simulink model "Impedance"  (R2020b)
settings: Solver=FixedStepAuto  StartTime=0.0  StopTime=5  FixedStep=0.005  RelTol=1e-3
values from neighbouring files (symbols this model uses):
  inv_Md = inv(Md)    [params.m]
  Kd = diag([30 30 14 1 1 1])    [params.m]
  Kp = diag([300 1000 300 1 1 1])    [params.m]
  Md = diag([1 0.1 1 1 1 1])    [params.m]
libraries: robotcorelib x1, vrlib x1
settings Model: Creator=andre  LastModifiedBy=filippo

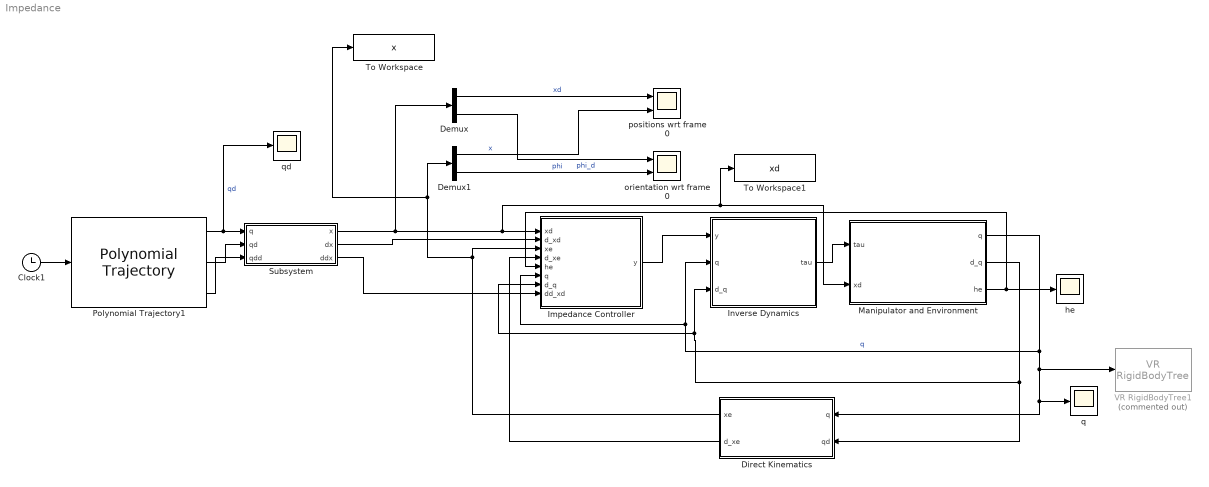
== system Impedance ==
  Clock1 : Clock
  Demux : Demux  Outputs=2
  Demux1 : Demux  Outputs=2
  Direct Kinematics : Subsystem
  Impedance Controller : Subsystem
  Inverse Dynamics : Subsystem
  Manipulator and Environment : Subsystem
  Polynomial Trajectory1 : robotcorelib/Polynomial Trajectory  WaypointSource=Internal  Waypoints=[0,0,0.05;0,0,-0.1;0,0.1,0.1]  TimePoints=[ 0, 2, 4 ]  TimeInterval=[ 1, 4 ]  Method=Cubic Polynomial  ParameterSource=Internal  VelocityBoundaryCondition=zeros(3,3)  AccelerationBoundaryCondition=zeros( 2, 5 )  SimulateUsing=Interpreted execution
  Subsystem : Subsystem
  To Workspace : ToWorkspace  VariableName=x  SaveFormat=Timeseries  SampleTime=-1
  To Workspace1 : ToWorkspace  VariableName=xd  SaveFormat=Timeseries  SampleTime=-1
  VR RigidBodyTree1 : vrlib/VR RigidBodyTree  Commented=on  RBT=robot  useRBT=on  Ts=-1  ForceViewerOpen=on
      settings: SourceProductBaseCode=SL
  he : Scope
  orientation wrt frame 0 : Scope  NumInputPorts=2
  positions wrt frame 0 : Scope  NumInputPorts=2
  q : Scope
  qd : Scope
  wires:
  Impedance Controller/1(y) -> Inverse Dynamics/1(y)
  Manipulator and Environment/2(d_q) -> Direct Kinematics/2(qd), Inverse Dynamics/3(d_q), Impedance Controller/7(d_q)
  Direct Kinematics/2(d_xe) -> Impedance Controller/4(d_xe)
  Manipulator and Environment/3(he) -> he/1, Impedance Controller/5(he)
  Direct Kinematics/1(xe) -> Impedance Controller/3(xe), To Workspace/1, Demux1/1
  Inverse Dynamics/1(tau) -> Manipulator and Environment/1(tau)
  Subsystem/1(x) -> Demux/1, To Workspace1/1, Manipulator and Environment/2(xd), Impedance Controller/1(xd)
  Subsystem/2(dx) -> Impedance Controller/2(d_xd)
  Polynomial Trajectory1/1 -> Subsystem/1(q), qd/1  "qd"
  Clock1/1 -> Polynomial Trajectory1/1
  Demux1/1 -> positions wrt frame 0/2  "x"
  Demux/1 -> positions wrt frame 0/1  "xd"
  Demux/2 -> orientation wrt frame 0/1  "phi_d"
  Demux1/2 -> orientation wrt frame 0/2  "phi"
  Manipulator and Environment/1(q) -> VR RigidBodyTree1/1, q/1, Direct Kinematics/1(q), Inverse Dynamics/2(q), Impedance Controller/6(q)  "q"
  Subsystem/3(ddx) -> Impedance Controller/8(dd_xd)
  Polynomial Trajectory1/2 -> Subsystem/2(qd)
  Polynomial Trajectory1/3 -> Subsystem/3(qdd)

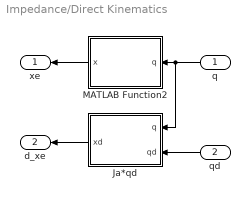
== system Impedance/Direct Kinematics ==
  q : Inport
  qd : Inport  Port=2
  Ja*qd : MATLAB Function  TreatAsAtomicUnit=on
  MATLAB Function2 : MATLAB Function  TreatAsAtomicUnit=on
  xe : Outport
  d_xe : Outport  Port=2
  wires:
  Ja*qd/1(xd) -> d_xe/1
  MATLAB Function2/1(x) -> xe/1
  q/1 -> Ja*qd/1(q), MATLAB Function2/1(q)
  qd/1 -> Ja*qd/2(qd)

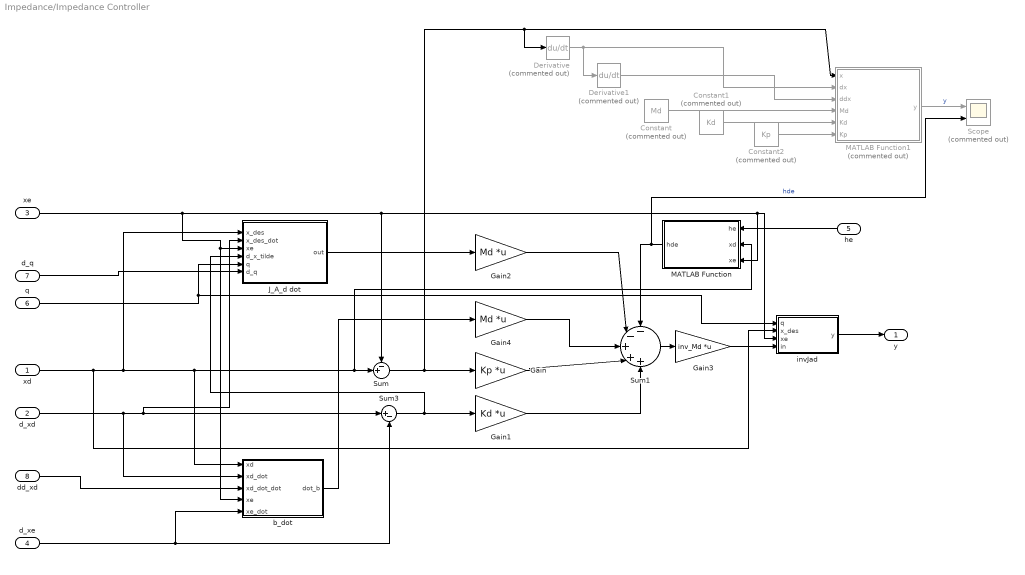
== system Impedance/Impedance Controller ==
  xd : Inport
  d_xd : Inport  Port=2
  xe : Inport  Port=3
  d_xe : Inport  Port=4
  he : Inport  Port=5
  q : Inport  Port=6
  d_q : Inport  Port=7
  dd_xd : Inport  Port=8
  Constant : Constant  Commented=on  Value=Md
  Constant1 : Constant  Commented=on  Value=Kd
  Constant2 : Constant  Commented=on  Value=Kp
  Derivative : Derivative  Commented=on
  Derivative1 : Derivative  Commented=on
  Gain : Gain  Gain=Kp  Multiplication=Matrix(K*u)
  Gain1 : Gain  Gain=Kd  Multiplication=Matrix(K*u)
  Gain2 : Gain  Gain=Md  Multiplication=Matrix(K*u)
  Gain3 : Gain  Gain=inv_Md  Multiplication=Matrix(K*u)
  Gain4 : Gain  Gain=Md  Multiplication=Matrix(K*u)
  J_A_d dot : MATLAB Function  TreatAsAtomicUnit=on
  MATLAB Function : MATLAB Function  TreatAsAtomicUnit=on
  MATLAB Function1 : MATLAB Function  Commented=on  TreatAsAtomicUnit=on
  Scope : Scope  Commented=on  NumInputPorts=2
  Sum : Sum  Inputs=-+|
  Sum1 : Sum  Inputs=-|-|+|+|+
  Sum3 : Sum  Inputs=|+-
  b_dot : MATLAB Function  TreatAsAtomicUnit=on
  invJad : MATLAB Function  TreatAsAtomicUnit=on
  y : Outport
  wires:
  xd/1 -> invJad/2(x_des), Sum/2, MATLAB Function/2(xd), b_dot/1(xd), J_A_d dot/1(x_des)
  xe/1 -> invJad/3(xe), MATLAB Function/3(xe), Sum/1, b_dot/4(xe), J_A_d dot/3(xe)
  Gain1/1 -> Sum1/5
  Gain/1 -> Sum1/4
  d_xe/1 -> b_dot/5(xe_dot), Sum3/2
  d_xd/1 -> b_dot/2(xd_dot), J_A_d dot/2(x_des_dot), Sum3/1
  Gain3/1 -> invJad/4(in)
  q/1 -> J_A_d dot/5(q), invJad/1(q)
  Sum1/1 -> Gain3/1
  he/1 -> MATLAB Function/1(he)
  MATLAB Function/1(hde) -> Scope/2, Sum1/1  "hde"
  Gain4/1 -> Sum1/3
  d_q/1 -> J_A_d dot/6(d_q)
  b_dot/1(dot_b) -> Gain4/1
  J_A_d dot/1(out) -> Gain2/1
  Gain2/1 -> Sum1/2
  invJad/1(y) -> y/1
  dd_xd/1 -> b_dot/3(xd_dot_dot)
  MATLAB Function1/1(y) -> Scope/1  "y"
  Constant/1 -> MATLAB Function1/4(Md)
  Constant1/1 -> MATLAB Function1/5(Kd)
  Constant2/1 -> MATLAB Function1/6(Kp)
  Sum/1 -> Derivative/1, MATLAB Function1/1(x), Gain/1
  Sum3/1 -> Gain1/1, J_A_d dot/4(d_x_tilde)
  Derivative/1 -> Derivative1/1, MATLAB Function1/2(dx)
  Derivative1/1 -> MATLAB Function1/3(ddx)

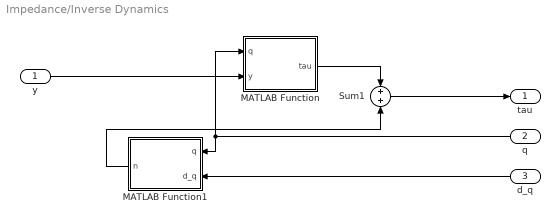
== system Impedance/Inverse Dynamics ==
  y : Inport
  q : Inport  Port=2
  d_q : Inport  Port=3
  MATLAB Function : MATLAB Function  TreatAsAtomicUnit=on
  MATLAB Function1 : MATLAB Function  TreatAsAtomicUnit=on
  Sum1 : Sum
  tau : Outport
  wires:
  MATLAB Function1/1(n) -> Sum1/2
  d_q/1 -> MATLAB Function1/2(d_q)
  q/1 -> MATLAB Function1/1(q), MATLAB Function/1(q)
  y/1 -> MATLAB Function/2(y)
  MATLAB Function/1(tau) -> Sum1/1
  Sum1/1 -> tau/1

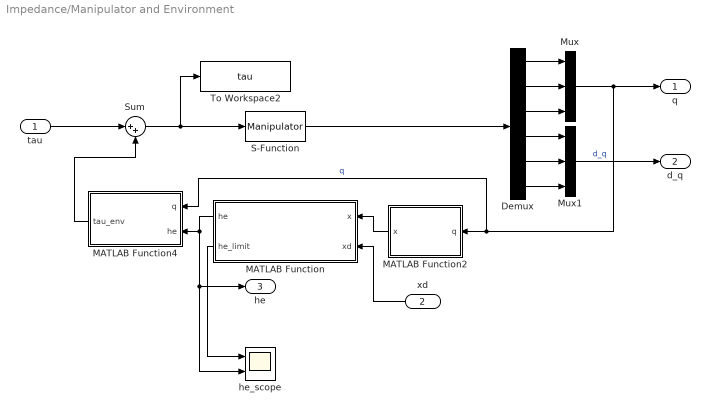
== system Impedance/Manipulator and Environment ==
  tau : Inport
  xd : Inport  Port=2
  Demux : Demux  Outputs=6
  MATLAB Function : MATLAB Function  TreatAsAtomicUnit=on
  MATLAB Function2 : MATLAB Function  TreatAsAtomicUnit=on
  MATLAB Function4 : MATLAB Function  TreatAsAtomicUnit=on
  Mux : Mux  Inputs=3
  Mux1 : Mux  Inputs=3
  S-Function : S-Function  FunctionName=Manipulator  Parameters=param  SFunctionDeploymentMode=off  EnableBusSupport=off
  Sum : Sum  Inputs=|++
  To Workspace2 : ToWorkspace  VariableName=tau  SaveFormat=Timeseries  SampleTime=-1
  he_scope : Scope  NumInputPorts=2
  q : Outport
  d_q : Outport  Port=2
  he : Outport  Port=3
  wires:
  Demux/4 -> Mux1/1
  tau/1 -> Sum/1
  Demux/3 -> Mux/3
  Demux/1 -> Mux/1
  Demux/5 -> Mux1/2
  Demux/6 -> Mux1/3
  Demux/2 -> Mux/2
  Mux1/1 -> d_q/1  "d_q"
  Mux/1 -> q/1, MATLAB Function4/1(q), MATLAB Function2/1(q)  "q"
  MATLAB Function2/1(x) -> MATLAB Function/1(x)
  S-Function/1 -> Demux/1
  Sum/1 -> To Workspace2/1, S-Function/1
  MATLAB Function/1(he) -> he_scope/2, he/1, MATLAB Function4/2(he)
  MATLAB Function4/1(tau_env) -> Sum/2
  MATLAB Function/2(he_limit) -> he_scope/1
  xd/1 -> MATLAB Function/2(xd)

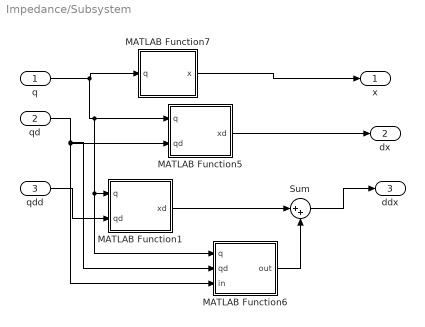
== system Impedance/Subsystem ==
  q : Inport
  qd : Inport  Port=2
  qdd : Inport  Port=3
  MATLAB Function1 : MATLAB Function  TreatAsAtomicUnit=on
  MATLAB Function5 : MATLAB Function  TreatAsAtomicUnit=on
  MATLAB Function6 : MATLAB Function  TreatAsAtomicUnit=on
  MATLAB Function7 : MATLAB Function  TreatAsAtomicUnit=on
  Sum : Sum  Inputs=|++
  x : Outport
  dx : Outport  Port=2
  ddx : Outport  Port=3
  wires:
  q/1 -> MATLAB Function6/1(q), MATLAB Function1/1(q), MATLAB Function5/1(q), MATLAB Function7/1(q)
  MATLAB Function7/1(x) -> x/1
  MATLAB Function5/1(xd) -> dx/1
  qdd/1 -> MATLAB Function1/2(qd)
  qd/1 -> MATLAB Function6/3(in), MATLAB Function5/2(qd), MATLAB Function6/2(qd)
  MATLAB Function6/1(out) -> Sum/2
  MATLAB Function1/1(xd) -> Sum/1
  Sum/1 -> ddx/1

== matlab function Impedance/Direct Kinematics/MATLAB Function2 ==
  data: q input; x output; param parameter
function x = Kin(q,param)
    x = Kinematics(q,param);
end

== matlab function Impedance/Direct Kinematics/Ja*qd ==
  data: q input; xd output; qd input; param parameter
function xd = Ja(q, qd, param)
    Ja = AnalyticalJacobian(q,param);
    xd = Ja * qd;
end

== matlab function Impedance/Impedance Controller/J_A_d dot ==
  data: x_des input; x_des_dot input; out output; xe input; d_x_tilde input; q input; d_q input; param parameter
function out = dot_Jad(x_des, x_des_dot, xe, d_x_tilde, q, d_q, param)    
    % Get euler angles from x_tilde
    x_tilde = x_des - xe;
    O_d_e = - x_tilde(4:6);
    phi = O_d_e(1);
    theta = O_d_e(2);
    
    % Get velocities along euler angles
    omega_d_e = - d_x_tilde(4:6);
    theta_dot = omega_d_e(1);
    phi_dot = omega_d_e(2);
    
    % Build rotation matrix
    Rd = eul2rotm(x_des(4:6)', 'ZYZ');
    R = [Rd', zeros(3,3); zeros(3,3), Rd'];
    
    % Get Ta and the necessary transformations
    Ta =  [1, 0, 0, 0, 0, 0;
            0, 1, 0, 0, 0, 0;
            0, 0, 1, 0, 0, 0;
            0, 0, 0, 0, -sin(phi), cos(phi) * sin(theta);
            0, 0, 0, 0, cos(phi), sin(phi) * sin(theta);
            0, 0, 0, 1, 0, cos(theta)];
    Ta_inv = pinv(Ta);
    
    % Precomputed dot inverse of Ta
    d_Ta = [[0, 0, 0, 0,                 0,                                                           0]
            [0, 0, 0, 0,                 0,                                                           0]
            [0, 0, 0, 0,                 0,                                                           0]
            [0, 0, 0, 0, -phi_dot*cos(phi), theta_dot*cos(phi)*cos(theta) - phi_dot*sin(phi)*sin(theta)]
            [0, 0, 0, 0, -phi_dot*sin(phi), phi_dot*cos(phi)*sin(theta) + theta_dot*cos(theta)*sin(phi)]
            [0, 0, 0, 0,                 0,                                       -theta_dot*sin(theta)]];
    Ta_inv_dot = pinv(d_Ta);
    
    % Build the skew symmetric matrix used to compute the derivative
    wd_d = x_des_dot(4:6);
    Swd = [   0      -wd_d(3)   wd_d(2);
              wd_d(3)       0      -wd_d(1);
             -wd_d(2)   wd_d(1)     0   ];
    
    % Compute the RS matrix with Rd' and the skew symmetric matrix
    RS = [Rd'*Swd, zeros(3,3); zeros(3,3), Rd'*Swd];
    
    % Jad = invTA*R*J
    dot_Jad = Ta_inv*(RS*Jacobian(q,param)+R*Jacobian_dot(q,d_q,param))+Ta_inv_dot*R*Jacobian(q,param);

    out = dot_Jad * d_q;
end

== matlab function Impedance/Impedance Controller/b_dot ==
  data: xd input; xd_dot input; xd_dot_dot input; dot_b output; xe input; xe_dot input
function dot_b = dot_b(xd, xd_dot, xd_dot_dot, xe, xe_dot)
    Rd = eul2rotm(xd(4:6)', 'ZYZ');
    
    % Get x_tilde and x_tilde_dot
    x_tilde = xd - xe;
    d_x_tilde = xd_dot - xe_dot;
    
    % Get angles from x_tilde
    phi_d_e = - x_tilde(4:6); 
    phi = phi_d_e(1);
    theta = phi_d_e(2);
    theta_dot = -d_x_tilde(2);
    phi_dot = -d_x_tilde(1);
    
    % Get the transformation matrix ZYZ
    T = [0   -sin(phi)  cos(phi)*sin(theta);
         0  cos(theta)  sin(phi)*sin(theta);
         1      0                cos(theta)];
    
    % Compute T_inv_dot
    d_T = [[0,     -phi_dot*cos(phi), theta_dot*cos(phi)*cos(theta) - phi_dot*sin(phi)*sin(theta)]
            [0, -theta_dot*sin(theta), phi_dot*cos(phi)*sin(theta) + theta_dot*cos(theta)*sin(phi)]
            [0,                     0,                                       -theta_dot*sin(theta)]];
    invT = pinv(T);
    invDT = -invT*d_T*invT;
            
    % Angular velocity and linearSwd_d velocity
    wd_d = xd_dot(4:6);
    dot_wd_d = xd_dot_dot(4:6);
    
    % Skew symmetric matrix
    Swd_d = [   0      -wd_d(3)   wd_d(2);
              wd_d(3)       0      -wd_d(1);
             -wd_d(2)   wd_d(1)     0   ];
    d_Rd = Rd'*Swd_d;
    
    % o d-e and its derivatives
    oe = xe(1:3);
    od = xd(1:3);
    dot_oe = xe_dot(1:3);
    dot_od = xd_dot(1:3);
    od_dot = xd_dot(1:3);
    od_dot_dot = xd_dot_dot(1:3);
    
    
    dot_b = [Rd'*od_dot_dot+d_Rd'*od_dot + cross(Rd'*dot_wd_d,Rd'*(od-oe)) + cross(Rd'*wd_d, Rd'*(dot_od-dot_oe));
        invDT*wd_d + invT*dot_wd_d];
end

== matlab function Impedance/Inverse Dynamics/MATLAB Function1 ==
  data: q input; n output; d_q input; param parameter
function n = n(q,d_q,param)
    % Compute C and G used in the model of n(q,d_q)
    C = double(C_Lagrangian(q, d_q, param));
    G = double(G_Lagrangian(q, param));
    Fsv = param.Fsv;

    n = C * d_q + G + Fsv * d_q;
end

== matlab function Impedance/Subsystem/MATLAB Function1 ==
  data: q input; qd input; xd output; param parameter
function xd = Ja(q, qd, param)
    Ja = AnalyticalJacobian(q,param);
    xd = Ja * qd;
end

== matlab function Impedance/Manipulator and Environment/MATLAB Function ==
  data: x input; xd input; he output; param parameter; he_limit output
function [he, he_limit] = environment(x, xd, param)
    if x(param.axis) >= param.wall 

        % set up the rest position frame
        xr = zeros(6,1);
        xr(param.axis) = param.wall;

        xe = zeros(6,1);
        xe(param.axis) = x(param.axis);

        he = param.K * (xe - xr);
        dx_rd = zeros(6,1);
        dx_rd(param.axis) = xd(param.axis) - xr(param.axis);
        % At the limit
        he_limit =  param.K/(eye(6) + param.K / param.Kp) * dx_rd;
    else
        he = zeros(6,1);
        he_limit = zeros(6,1);
    end
end

== matlab function Impedance/Manipulator and Environment/MATLAB Function2 ==
  data: q input; x output; param parameter
function x = Kin(q,param)
    x = Kinematics(q,param);
end

== matlab function Impedance/Subsystem/MATLAB Function5 ==
  data: q input; qd input; xd output; param parameter
function xd = Ja(q, qd, param)
    Ja = AnalyticalJacobian(q,param);
    xd = Ja * qd;
end

== matlab function Impedance/Subsystem/MATLAB Function6 ==
  data: q input; qd input; in input; out output; param parameter
function out = dot_Ja(q, qd, in, param)
    d_Ja = AnalyticalJacobian_dot(q,qd,param);
    out = d_Ja * in;
end

== matlab function Impedance/Subsystem/MATLAB Function7 ==
  data: q input; x output; param parameter
function x = Kin(q,param)
    x = Kinematics(q,param);
end

== matlab function Impedance/Manipulator and Environment/MATLAB Function4 ==
  data: q input; he input; tau_env output; param parameter
function tau_env = JT(q, he, param)
    tau_env = -Jacobian(q, param)' * he;
end

== matlab function Impedance/Impedance Controller/MATLAB Function1 ==
  data: x input; y output; dx input; ddx input; Md input; Kd input; Kp input
function y = eq(x, dx, ddx, Md, Kd, Kp)
    y = Md*ddx + Kd*dx + Kp*x;

== matlab function Impedance/Inverse Dynamics/MATLAB Function ==
  data: q input; y input; tau output; param parameter
function tau = B(q,y,param)
    B_matrix = B_Lagrangian(q, param);
    tau =  B_matrix * y;
end

== matlab function Impedance/Impedance Controller/invJad ==
  data: q input; x_des input; xe input; y output; in input; param parameter
function y = invJad(q, x_des, xe, in, param)
    x_tilde = x_des - xe;
    Rd = eul2rotm(-x_tilde(4:6)','ZYZ');
    angles = -x_tilde(4:6);
    
%     Compute Ta(phi_de) in this case ZYZ
    ph = -angles(1);
    th = -angles(2);
    Ta =   [1, 0, 0, 0, 0, 0;
            0, 1, 0, 0, 0, 0;
            0, 0, 1, 0, 0, 0;
            0, 0, 0, 0, -sin(ph), cos(ph) * sin(th);
            0, 0, 0, 0, cos(ph), sin(ph) * sin(th);
            0, 0, 0, 1, 0, cos(th)];
        
    Jad = pinv(Ta)*[Rd', zeros(3,3); zeros(3,3), Rd']*Jacobian(q, param);
 
    %Jad = AnalyticalJacobian(q,param);
     
    y = pinv(Jad) * in;
end

== matlab function Impedance/Impedance Controller/MATLAB Function ==
  data: he input; hde output; xd input; xe input
function hde = to_hde(he, xd, xe)
    hde = zeros(6,1);
    Rd_e = eul2rotm(((xd(4:6) - xe(4:6)))', 'ZYZ');
    
    hde(1:3) = Rd_e * he(1:3);
    hde(4:6) = Rd_e * he(4:6);
end
